simulink model "find_T"  (R2021a)
settings: Solver=VariableStepAuto  StartTime=0.0  StopTime=10.0  RelTol=1e-3
undefined symbols (not defined in the file): A, C, F, L
settings Model: Creator=ASUS  LastModifiedBy=ASUS

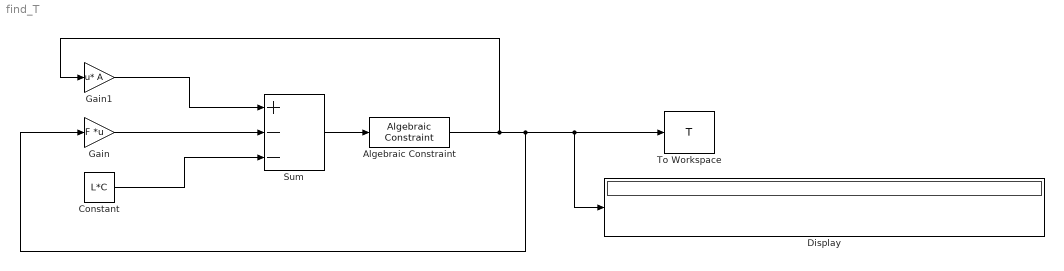
== system find_T ==
  Algebraic Constraint : AlgebraicConstraint
  Constant : Constant  Value=L*C
  Display : Display
  Gain : Gain  Gain=F  Multiplication=Matrix(K*u)
  Gain1 : Gain  Gain=A  Multiplication=Matrix(u*K)
  Sum : Sum  Inputs=+--
  To Workspace : ToWorkspace  VariableName=T  SampleTime=-1
      settings: MaxDataPoints=3  Save2DSignal=2-D array (concatenate along first dimension)
  wires:
  Sum/1 -> Algebraic Constraint/1
  Algebraic Constraint/1 -> Gain1/1, Gain/1, Display/1, To Workspace/1
  Constant/1 -> Sum/3
  Gain/1 -> Sum/2
  Gain1/1 -> Sum/1
